simulink model "AER3640_avion_wind"  (R2025a)
settings: Solver=VariableStepAuto  StartTime=0.0  StopTime=100  RelTol=1e-3  EnableMultiTasking=on
values from neighbouring files (symbols this model uses):
  V_w = zeros(size(t_sim))    [validation_laboratoire_5.m]
undefined symbols (not defined in the file or in its folder): conditions, model
settings Model: Creator=Georges  LastModifiedBy=lambe
settings SolverCC: AlgebraicLoopSolver=TrustRegion
settings DataIOCC: LimitDataPoints=on  ReturnWorkspaceOutputs=off
settings OptimizationCC: LifeSpan=inf
settings DebuggingCC: UnconnectedInputMsg=warning  UnconnectedOutputMsg=warning  UnconnectedLineMsg=warning  AllowSymbolicDim=off  SFUnexpectedBacktrackingDiag=warning  SFNoUnconditionalDefaultTransitionDiag=warning  SFExecutionAtInitializationDiag=none  ArithmeticOperatorsInVariantConditions=warning
settings ModelReferenceCC: EnableRefExpFcnMdlSchedulingChecks=on  PropagateSignalLabelsOutOfModel=off
settings SFSimCC: SimUseLocalCustomCode=off  CustomCodeUndefinedFunction=UseInterfaceOnly
settings RTWCC: RTWUseLocalCustomCode=off  GPUComputeCapability=3.5
settings CodeAppCC: StateflowObjectComments=on
settings GRTTargetCC: TargetLangStandard=C89/C90 (ANSI)
settings ConfigComp: CovMetricSettings=dw  CovSaveCumulativeToWorkspaceVar=on  CovSaveSingleToWorkspaceVar=on  CovExternalEMLEnable=off

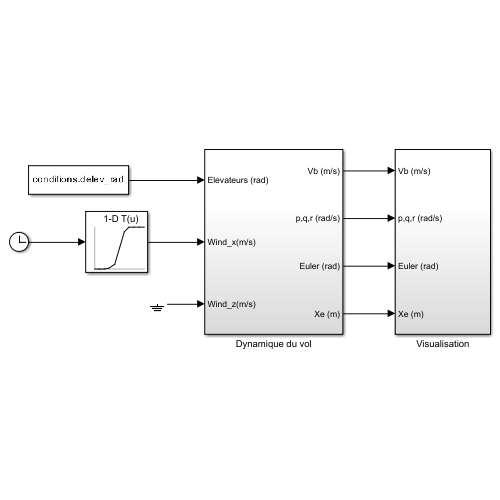
[thumbnail: Simulink's stored preview of the top-level diagram]
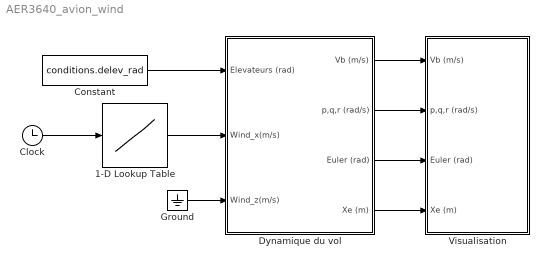
== system AER3640_avion_wind ==
  1-D Lookup Table : Lookup_n-D  NumberOfTableDimensions=1  LookupTableObject=V_w  BreakpointsForDimension1=[0:0.1:300]  Table=V_w  InternalRulePriority=Speed  RndMeth=Simplest
  Clock : Clock
  Constant : Constant  Value=conditions.delev_rad
  Dynamique du vol : Subsystem
  Ground : Ground
  Visualisation : Subsystem
  wires:
  Dynamique du vol/1(Vb (m/s)) -> Visualisation/1(Vb (m/s))
  Dynamique du vol/4(Xe (m)) -> Visualisation/4(Xe (m))
  Dynamique du vol/2(p,q,r (rad/s)) -> Visualisation/2(p,q,r (rad/s))
  Dynamique du vol/3(Euler (rad)) -> Visualisation/3(Euler (rad))
  Ground/1 -> Dynamique du vol/3(Wind_z(m/s))
  Constant/1 -> Dynamique du vol/1(Elevateurs (rad))
  1-D Lookup Table/1 -> Dynamique du vol/2(Wind_x(m/s))
  Clock/1 -> 1-D Lookup Table/1

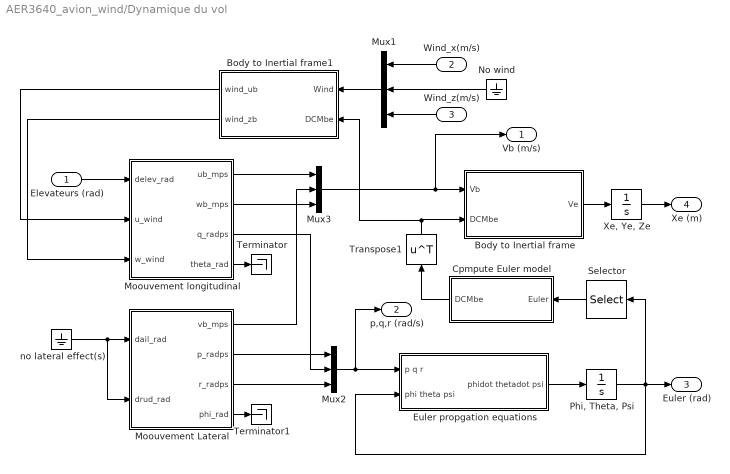
== system AER3640_avion_wind/Dynamique du vol ==
  Elevateurs (rad) : Inport
  Wind_x(m/s) : Inport  Port=2
  Wind_z(m/s) : Inport  Port=3
  Body to Inertial frame : Subsystem
  Body to Inertial frame1 : Subsystem
  Cpmpute Euler model : Subsystem
  Euler propgation equations : Subsystem
  Moouvement Lateral : Subsystem
  Moouvement longitudinal : Subsystem
  Mux1 : Mux  Inputs=3
  Mux2 : Mux  Inputs=3
  Mux3 : Mux  Inputs=3
  No wind : Ground
  "Phi, Theta, Psi" : Integrator  InitialCondition=[0 conditions.theta_rad 0]
  Selector : Selector  InputPortWidth=3  IndexOptions=Index vector (dialog)  Indices=[3 2 1]  OutputSizes=1
  Terminator : Terminator
  Terminator1 : Terminator
  Transpose1 : Math  Operator=transpose  SignedPower=on
  "Xe, Ye, Ze" : Integrator  InitialCondition=[0,0 -conditions.altitude_m]
  no lateral effect(s) : Ground
  Vb (m/s) : Outport
  p,q,r (rad/s) : Outport  Port=2
  Euler (rad) : Outport  Port=3
  Xe (m) : Outport  Port=4
  wires:
  Elevateurs (rad)/1 -> Moouvement longitudinal/1(delev_rad)
  no lateral effect(s)/1 -> Moouvement Lateral/2(drud_rad), Moouvement Lateral/1(dail_rad)
  "Phi, Theta, Psi"/1 -> Selector/1, Euler (rad)/1, Euler propgation equations/2(phi theta psi)
  Euler propgation equations/1(phidot thetadot psi) -> "Phi, Theta, Psi"/1
  Moouvement longitudinal/1(ub_mps) -> Mux3/1
  Moouvement longitudinal/2(wb_mps) -> Mux3/3
  Moouvement Lateral/1(vb_mps) -> Mux3/2
  Moouvement Lateral/3(r_radps) -> Mux2/3
  Moouvement Lateral/2(p_radps) -> Mux2/1
  Moouvement longitudinal/3(q_radps) -> Mux2/2
  Cpmpute Euler model/1(DCMbe) -> Transpose1/1
  Body to Inertial frame/1(Ve) -> "Xe, Ye, Ze"/1
  "Xe, Ye, Ze"/1 -> Xe (m)/1
  Mux3/1 -> Body to Inertial frame/1(Vb), Vb (m/s)/1
  Mux2/1 -> Euler propgation equations/1(p q r), p,q,r (rad/s)/1
  Transpose1/1 -> Body to Inertial frame1/2(DCMbe), Body to Inertial frame/2(DCMbe)
  Selector/1 -> Cpmpute Euler model/1(Euler)
  Moouvement longitudinal/4(theta_rad) -> Terminator/1
  Moouvement Lateral/4(phi_rad) -> Terminator1/1
  Mux1/1 -> Body to Inertial frame1/1(Wind)
  No wind/1 -> Mux1/2
  Body to Inertial frame1/1(wind_ub) -> Moouvement longitudinal/2(u_wind)
  Body to Inertial frame1/2(wind_zb) -> Moouvement longitudinal/3(w_wind)
  Wind_x(m/s)/1 -> Mux1/1
  Wind_z(m/s)/1 -> Mux1/3

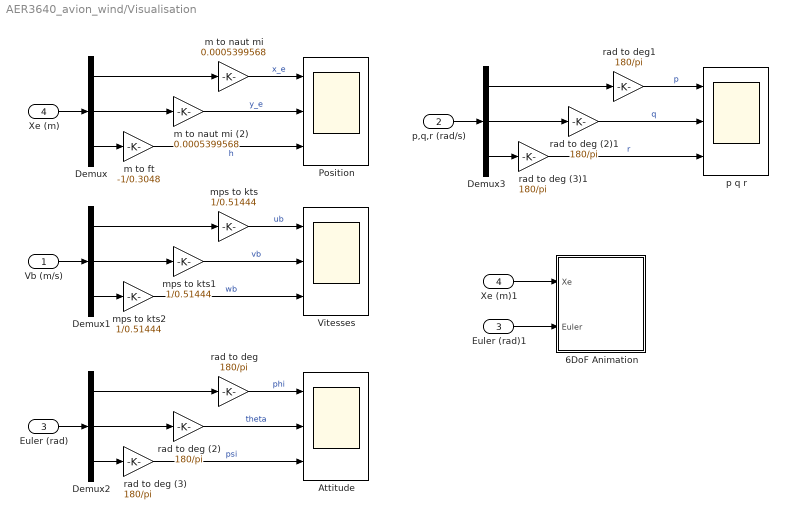
== system AER3640_avion_wind/Visualisation ==
  Vb (m/s) : Inport
  p,q,r (rad/s) : Inport  Port=2
  Euler (rad) : Inport  Port=3
  Xe (m) : Inport  Port=4
  6DoF Animation : Subsystem  mask(6DoF_Animation){u1=[0 4000 -2000 2000 -5000 -3000], u2=0.5, u3=50, u4=[0 0 0], u5=Fly alongside, u6=[75 25 -15], u7=50, u8=on}
      mask prompts: u1 "Axes limits [xmin xmax ymix ymax]:"; u2 "Time interval between updates:"; u3 "Size of craft displayed:"; u4 "Static object position [xp yp zp]:"; u5 "Enter view:"; u6 "Position of camera [xc yc zc]"; u7 "View angle"; u8 "Enable animation"
      mask init:
      | Config.axes = u1;
      | Config.update = u2;
      | Config.craft = u3;
      | Config.target = u4;
      | Config.camera_view = u5;
      | Config.camera_pos = u6;
      | Config.view = u7;
      | Config.Animenable = u8;
      | Config.Model = bdroot(gcb);
      mask TypeOptions u5: Fixed position | Cockpit | Fly alongside
  Attitude : Scope  NumInputPorts=3
      settings: ActiveDisplayYMinimum=-1  ActiveDisplayYMaximum=1  DataLoggingVariableName=euler
  Demux{,1..3} (4 alike) : Demux  Outputs=3
  Euler (rad)1 : InportShadow  Port=3
  Position : Scope  NumInputPorts=3
      settings: ActiveDisplayYMinimum=-0.87491  ActiveDisplayYMaximum=7.87419  DataLoggingVariableName=positions
  Vitesses : Scope  NumInputPorts=3
      settings: ActiveDisplayYMinimum=243.15212  ActiveDisplayYMaximum=261.72404  DataLoggingVariableName=vitesses
  Xe (m)1 : InportShadow  Port=4
  m to ft : Gain  Gain=-1/0.3048
  m to naut mi : Gain  Gain=0.0005399568
  m to naut mi (2) : Gain  Gain=0.0005399568
  mps to kts : Gain  Gain=1/0.51444
  mps to kts1 : Gain  Gain=1/0.51444
  mps to kts2 : Gain  Gain=1/0.51444
  p q r : Scope  NumInputPorts=3
      settings: ActiveDisplayYMinimum=-1  ActiveDisplayYMaximum=1  DataLoggingVariableName=pqr
  rad to deg : Gain  Gain=180/pi
  rad to deg (2) : Gain  Gain=180/pi
  rad to deg (2)1 : Gain  Gain=180/pi
  rad to deg (3) : Gain  Gain=180/pi
  rad to deg (3)1 : Gain  Gain=180/pi
  rad to deg1 : Gain  Gain=180/pi
  wires:
  Xe (m)/1 -> Demux/1
  Demux/1 -> m to naut mi/1
  Demux/2 -> m to naut mi (2)/1
  Demux/3 -> m to ft/1
  m to ft/1 -> Position/3  "h"
  m to naut mi (2)/1 -> Position/2  "y_e"
  m to naut mi/1 -> Position/1  "x_e"
  Xe (m)1/1 -> 6DoF Animation/1(Xe)
  Euler (rad)1/1 -> 6DoF Animation/2(Euler)
  Vb (m/s)/1 -> Demux1/1
  Demux1/2 -> mps to kts1/1
  Demux1/1 -> mps to kts/1
  Demux1/3 -> mps to kts2/1
  mps to kts/1 -> Vitesses/1  "ub"
  mps to kts1/1 -> Vitesses/2  "vb"
  mps to kts2/1 -> Vitesses/3  "wb"
  Euler (rad)/1 -> Demux2/1
  Demux2/2 -> rad to deg (2)/1
  Demux2/1 -> rad to deg/1
  Demux2/3 -> rad to deg (3)/1
  rad to deg/1 -> Attitude/1  "phi"
  rad to deg (2)/1 -> Attitude/2  "theta"
  rad to deg (3)/1 -> Attitude/3  "psi"
  p,q,r (rad/s)/1 -> Demux3/1
  Demux3/2 -> rad to deg (2)1/1
  Demux3/1 -> rad to deg1/1
  Demux3/3 -> rad to deg (3)1/1
  rad to deg1/1 -> p q r/1  "p"
  rad to deg (2)1/1 -> p q r/2  "q"
  rad to deg (3)1/1 -> p q r/3  "r"

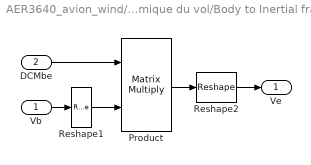
== system AER3640_avion_wind/Dynamique du vol/Body to Inertial frame ==
  Vb : Inport
  DCMbe : Inport  Port=2
  Product : Product  Multiplication=Matrix(*)  InputSameDT=on  SaturateOnIntegerOverflow=on  OutDataTypeStr=Inherit: Same as first input
  Reshape1 : Reshape  OutputDimensionality=Column vector (2-D)
  Reshape2 : Reshape
  Ve : Outport
  wires:
  Product/1 -> Reshape2/1
  Reshape2/1 -> Ve/1
  Vb/1 -> Reshape1/1
  Reshape1/1 -> Product/2
  DCMbe/1 -> Product/1

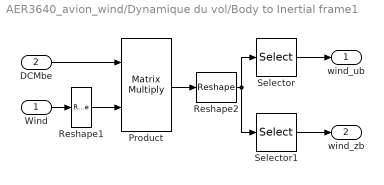
== system AER3640_avion_wind/Dynamique du vol/Body to Inertial frame1 ==
  Wind : Inport
  DCMbe : Inport  Port=2
  Product : Product  Multiplication=Matrix(*)  InputSameDT=on  SaturateOnIntegerOverflow=on  OutDataTypeStr=Inherit: Same as first input
  Reshape1 : Reshape  OutputDimensionality=Column vector (2-D)
  Reshape2 : Reshape
  Selector : Selector  InputPortWidth=3  IndexOptions=Index vector (dialog)  Indices=1  OutputSizes=1
  Selector1 : Selector  InputPortWidth=3  IndexOptions=Index vector (dialog)  Indices=3  OutputSizes=1
  wind_ub : Outport
  wind_zb : Outport  Port=2
  wires:
  DCMbe/1 -> Product/1
  Reshape1/1 -> Product/2
  Wind/1 -> Reshape1/1
  Product/1 -> Reshape2/1
  Reshape2/1 -> Selector1/1, Selector/1
  Selector/1 -> wind_ub/1
  Selector1/1 -> wind_zb/1

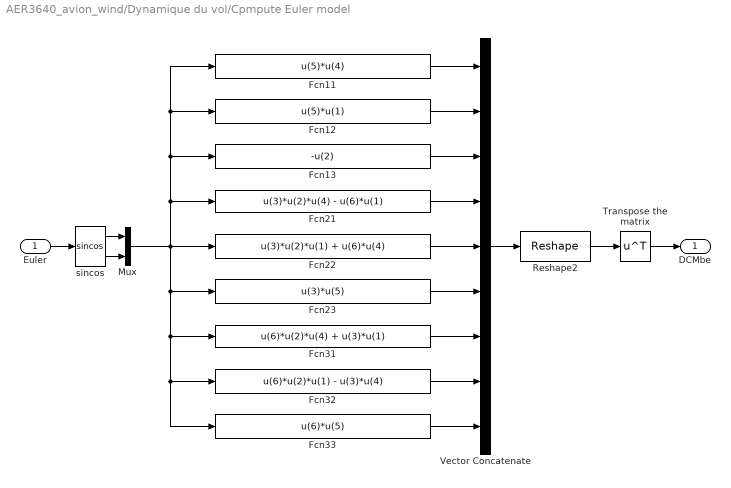
== system AER3640_avion_wind/Dynamique du vol/Cpmpute Euler model ==
  Euler : Inport
  Fcn11 : Fcn  Expr=u(5)*u(4)
  Fcn12 : Fcn  Expr=u(5)*u(1)
  Fcn13 : Fcn  Expr=-u(2)
  Fcn21 : Fcn  Expr=u(3)*u(2)*u(4) - u(6)*u(1)
  Fcn22 : Fcn  Expr=u(3)*u(2)*u(1) + u(6)*u(4)
  Fcn23 : Fcn  Expr=u(3)*u(5)
  Fcn31 : Fcn  Expr=u(6)*u(2)*u(4) + u(3)*u(1)
  Fcn32 : Fcn  Expr=u(6)*u(2)*u(1) - u(3)*u(4)
  Fcn33 : Fcn  Expr=u(6)*u(5)
  Mux : Mux  Inputs=2
  Reshape2 : Reshape  OutputDimensionality=Customize  OutputDimensions=[3,3]
  Transpose the matrix : Math  Operator=transpose  SignedPower=on
  Vector Concatenate : Concatenate  NumInputs=9
  sincos : Trigonometry  Operator=sincos
  DCMbe : Outport
  wires:
  Euler/1 -> sincos/1
  sincos/1 -> Mux/1
  sincos/2 -> Mux/2
  Mux/1 -> Fcn22/1, Fcn21/1, Fcn13/1, Fcn11/1, Fcn12/1, Fcn23/1, Fcn31/1, Fcn33/1, Fcn32/1
  Vector Concatenate/1 -> Reshape2/1
  Fcn23/1 -> Vector Concatenate/6
  Fcn22/1 -> Vector Concatenate/5
  Fcn31/1 -> Vector Concatenate/7
  Fcn21/1 -> Vector Concatenate/4
  Fcn32/1 -> Vector Concatenate/8
  Fcn33/1 -> Vector Concatenate/9
  Fcn13/1 -> Vector Concatenate/3
  Fcn12/1 -> Vector Concatenate/2
  Fcn11/1 -> Vector Concatenate/1
  Reshape2/1 -> Transpose the matrix/1
  Transpose the matrix/1 -> DCMbe/1

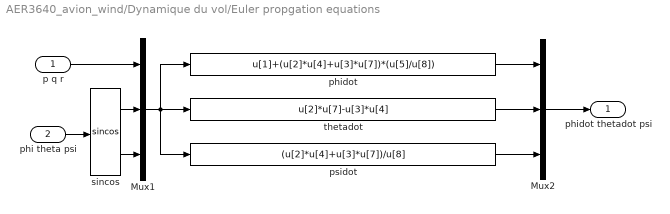
== system AER3640_avion_wind/Dynamique du vol/Euler propgation equations ==
  p q r : Inport
  phi theta psi : Inport  Port=2
  Mux1 : Mux  Inputs=[3 3 3]
  Mux2 : Mux  Inputs=3
  phidot : Fcn  Expr=u[1]+(u[2]*u[4]+u[3]*u[7])*(u[5]/u[8])
  psidot : Fcn  Expr=(u[2]*u[4]+u[3]*u[7])/u[8]
  sincos : Trigonometry  Operator=sincos
  thetadot : Fcn  Expr=u[2]*u[7]-u[3]*u[4]
  phidot thetadot psi : Outport  InitialOutput=0
  wires:
  Mux1/1 -> psidot/1, phidot/1, thetadot/1
  p q r/1 -> Mux1/1
  phi theta psi/1 -> sincos/1
  psidot/1 -> Mux2/3
  thetadot/1 -> Mux2/2
  phidot/1 -> Mux2/1
  Mux2/1 -> phidot thetadot psi/1
  sincos/1 -> Mux1/2
  sincos/2 -> Mux1/3

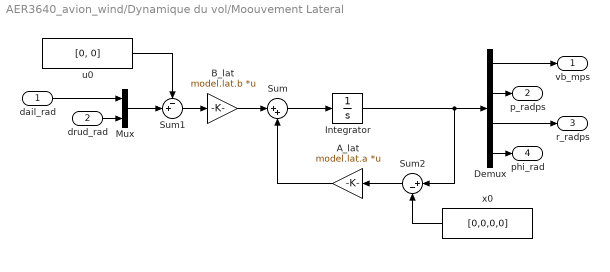
== system AER3640_avion_wind/Dynamique du vol/Moouvement Lateral ==
  dail_rad : Inport
  drud_rad : Inport  Port=2
  A_lat : Gain  Gain=model.lat.a  Multiplication=Matrix(K*u) (u vector)
  B_lat : Gain  Gain=model.lat.b  Multiplication=Matrix(K*u) (u vector)
  Demux : Demux
  Integrator : Integrator
  Mux : Mux  Inputs=2
  Sum : Sum  Inputs=|++
  Sum1 : Sum  Inputs=-+|
  Sum2 : Sum  Inputs=|+-
  u0 : Constant  Value=[0, 0]
  x0 : Constant  Value=[0,0,0,0]
  vb_mps : Outport
  p_radps : Outport  Port=2
  r_radps : Outport  Port=3
  phi_rad : Outport  Port=4
  wires:
  Demux/2 -> p_radps/1
  Demux/3 -> r_radps/1
  Demux/4 -> phi_rad/1
  Demux/1 -> vb_mps/1
  drud_rad/1 -> Mux/2
  dail_rad/1 -> Mux/1
  Mux/1 -> Sum1/2
  Sum/1 -> Integrator/1
  A_lat/1 -> Sum/2
  B_lat/1 -> Sum/1
  u0/1 -> Sum1/1
  Sum1/1 -> B_lat/1
  Sum2/1 -> A_lat/1
  x0/1 -> Sum2/2
  Integrator/1 -> Demux/1, Sum2/1

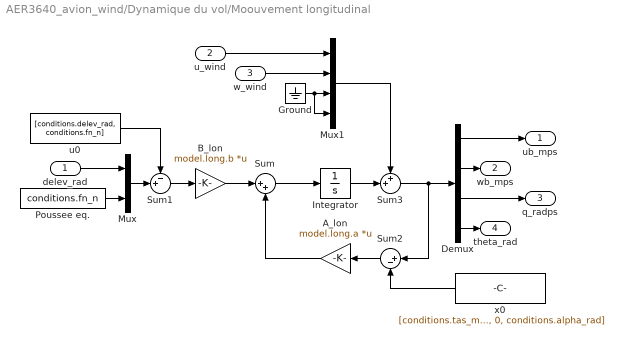
== system AER3640_avion_wind/Dynamique du vol/Moouvement longitudinal ==
  delev_rad : Inport
  u_wind : Inport  Port=2
  w_wind : Inport  Port=3
  A_lon : Gain  Gain=model.long.a  Multiplication=Matrix(K*u) (u vector)
  B_lon : Gain  Gain=model.long.b  Multiplication=Matrix(K*u) (u vector)
  Demux : Demux
  Ground : Ground
  Integrator : Integrator  InitialCondition=[conditions.tas_mps*cos(conditions.alpha_rad), conditions.tas_mps*sin(conditions.alpha_rad), 0, conditions.alpha_rad]
  Mux : Mux  Inputs=2
  Mux1 : Mux
  Poussee eq. : Constant  Value=conditions.fn_n
  Sum : Sum  Inputs=|++
  Sum1 : Sum  Inputs=-+|
  Sum2 : Sum  Inputs=|+-
  Sum3 : Sum  Inputs=++|
  u0 : Constant  Value=[conditions.delev_rad, conditions.fn_n]
  x0 : Constant  Value=[conditions.tas_mps*cos(conditions.alpha_rad), conditions.tas_mps*sin(conditions.alpha_rad), 0, conditions.alpha_rad]
  ub_mps : Outport
  wb_mps : Outport  Port=2
  q_radps : Outport  Port=3
  theta_rad : Outport  Port=4
  wires:
  Sum1/1 -> B_lon/1
  u0/1 -> Sum1/1
  B_lon/1 -> Sum/1
  A_lon/1 -> Sum/2
  Sum/1 -> Integrator/1
  Mux/1 -> Sum1/2
  delev_rad/1 -> Mux/1
  Poussee eq./1 -> Mux/2
  Demux/1 -> ub_mps/1
  Demux/4 -> theta_rad/1
  Demux/3 -> q_radps/1
  Demux/2 -> wb_mps/1
  Sum2/1 -> A_lon/1
  x0/1 -> Sum2/2
  Integrator/1 -> Sum3/2
  Sum3/1 -> Sum2/1, Demux/1
  Mux1/1 -> Sum3/1
  Ground/1 -> Mux1/4, Mux1/3
  u_wind/1 -> Mux1/1
  w_wind/1 -> Mux1/2

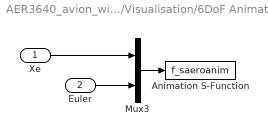
== system AER3640_avion_wind/Visualisation/6DoF Animation ==
  Xe : Inport
  Euler : Inport  Port=2
  Animation S-Function : S-Function  FunctionName=f_saeroanim  Parameters=Config  SFunctionDeploymentMode=off  EnableBusSupport=off
  Mux3 : Mux  Inputs=2
  wires:
  Mux3/1 -> Animation S-Function/1
  Euler/1 -> Mux3/2
  Xe/1 -> Mux3/1
